simulink model "Skateboard_Suspension_Half_Board_Model_2_Simulink"  (R2022b)
settings: Solver=VariableStepAuto  StartTime=0.0  StopTime=10.0  RelTol=1e-3
undefined symbols (not defined in the file): cF2, cw, kF1, kw, mbt, md, mtt
settings Model: Creator=victo  LastModifiedBy=victo

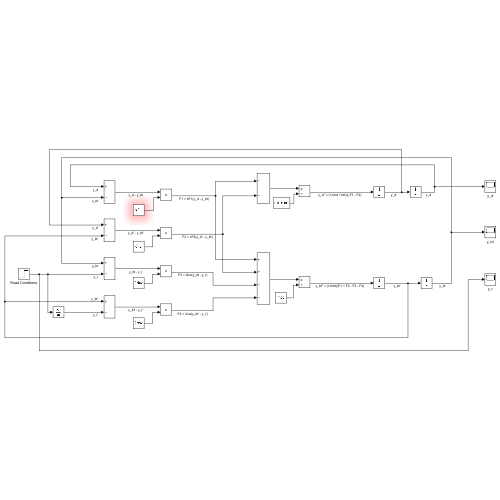
[thumbnail: Simulink's stored preview of the top-level diagram]
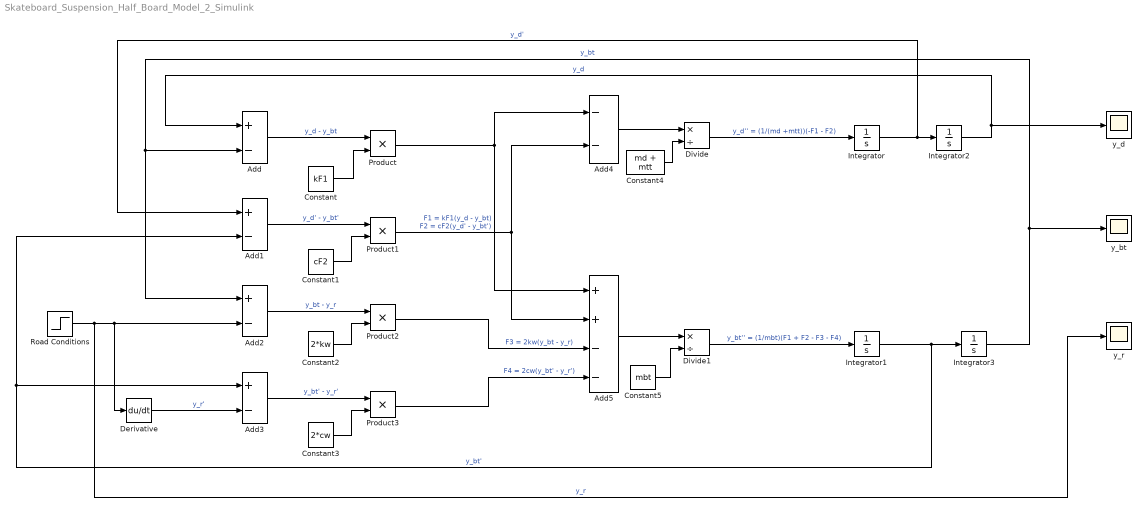
== system Skateboard_Suspension_Half_Board_Model_2_Simulink ==
  Add{,1..3} (4 alike) : Sum  Inputs=+-
  Add4 : Sum  Inputs=--
  Add5 : Sum  Inputs=++--
  Constant : Constant  Value=kF1
  Constant1 : Constant  Value=cF2
  Constant2 : Constant  Value=2*kw
  Constant3 : Constant  Value=2*cw
  Constant4 : Constant  Value=md + mtt
  Constant5 : Constant  Value=mbt
  Derivative : Derivative
  Divide : Product  Inputs=*/
  Divide1 : Product  Inputs=*/
  Integrator{,1..3} (4 alike) : Integrator
  Product{,1..3} (4 alike) : Product
  Road Conditions : Step  SampleTime=0
  y_bt : Scope
  y_d : Scope
  y_r : Scope
  wires:
  Integrator/1 -> Add1/1, Integrator2/1  "y_d'"
  Integrator3/1 -> y_bt/1, Add2/1, Add/2  "y_bt"
  Road Conditions/1 -> y_r/1, Derivative/1, Add2/2  "y_r"
  Integrator1/1 -> Add3/1, Add1/2, Integrator3/1  "y_bt'"
  Derivative/1 -> Add3/2  "y_r'"
  Add/1 -> Product/1  "y_d - y_bt"
  Add1/1 -> Product1/1  "y_d' - y_bt'"
  Add2/1 -> Product2/1  "y_bt - y_r"
  Add3/1 -> Product3/1  "y_bt' - y_r'"
  Constant/1 -> Product/2
  Product/1 -> Add5/1, Add4/1  "F1 = kF1(y_d - y_bt)"
  Product1/1 -> Add5/2, Add4/2  "F2 = cF2(y_d' - y_bt')"
  Constant1/1 -> Product1/2
  Constant2/1 -> Product2/2
  Product2/1 -> Add5/3  "F3 = 2kw(y_bt - y_r)"
  Constant3/1 -> Product3/2
  Product3/1 -> Add5/4  "F4 = 2cw(y_bt' - y_r')"
  Add4/1 -> Divide/1
  Add5/1 -> Divide1/1
  Constant4/1 -> Divide/2
  Constant5/1 -> Divide1/2
  Divide/1 -> Integrator/1  "y_d'' = (1/(md +mtt))(-F1 - F2)"
  Divide1/1 -> Integrator1/1  "y_bt'' = (1/mbt)(F1 + F2 - F3 - F4)"
  Integrator2/1 -> Add/1, y_d/1  "y_d"
